simulink model "softLog"  (R2025b)
settings: configuration reference "MCConfiguration" (kept outside this file)
settings Model: DataDictionary=embeddedBoard_common.sldd  OrderFunctionsByDependency=on  Creator=rpumpo  LastModifiedBy=rpumpo
settings ConfigSetRef: SourceName=MCConfiguration

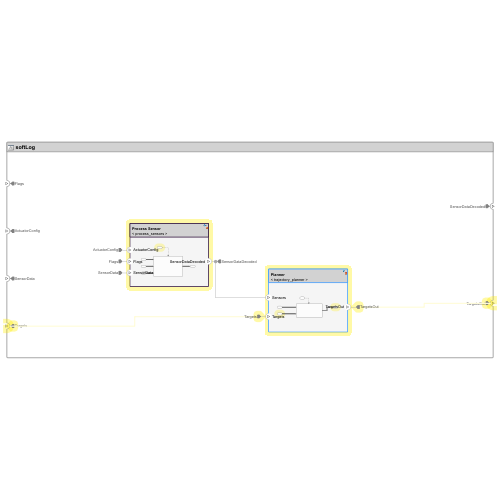
[thumbnail: Simulink's stored preview of the top-level diagram]
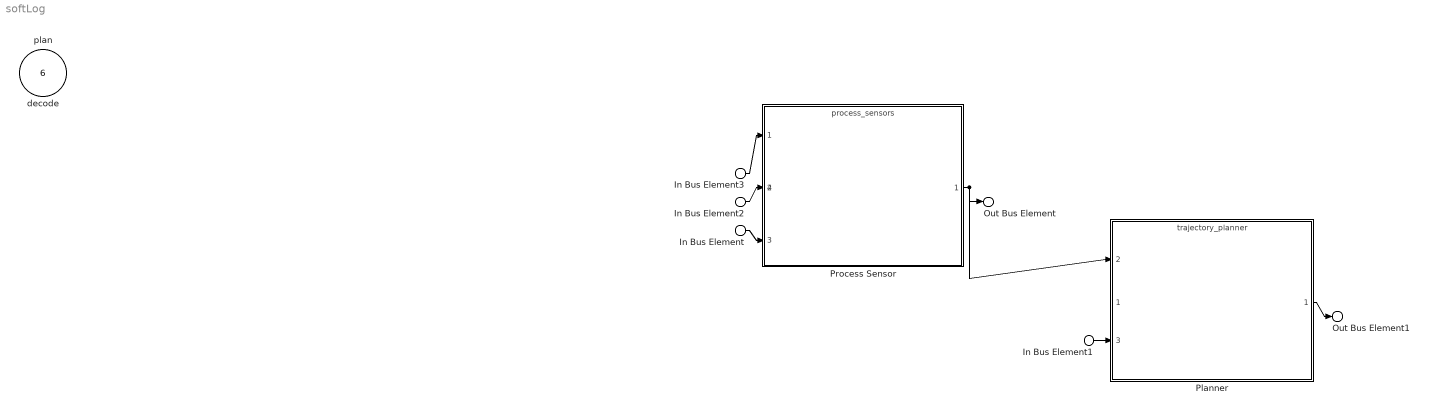
== system softLog ==
  In Bus Element2 : Inport  PortName=Flags
  In Bus Element3 : Inport  Port=2  PortName=ActuatorConfig
  In Bus Element : Inport  Port=3  PortName=SensorData
  In Bus Element1 : Inport  Port=4  PortName=Targets
  decode : Inport  Port=5  OutputFunctionCall=on
  plan : Inport  Port=6  OutputFunctionCall=on
  Planner : ModelReference  ModelNameDialog=trajectory_planner.slx  SimulationMode=Normal  ScheduleRates=on  ModelReferenceVersion=2.99
      settings: PortSchema="{\"entries\":[{\"content\":{\"headerSize\":38,\"margin\":15,\"minimumSpacing\":25,\"sides\":[{\"content\":{\"connectorIds\":[\"In2\",\"In3\"]},\"type\":\"ConnectorPlacement.EquallySpacedRectSide\",\"uuid\":\"5bc97249-f5b2-494b-970a-de3b3bfd1883\"},{\"content\":{\"connectorIds\":[\"Out1\"],\"side\":\"RIGHT\"},\"type\":\"ConnectorPlacement.EquallySpacedRectSide\",\"uuid\":\"c27ffe8a-4f1e-4977-8b42-d9f4b26c99eb\"},{\"content\":{\"side\":\"TOP\"},\"type\":\"ConnectorPlacement.EquallySpacedRectSide\",\"uuid\":\"ea9c3efe-70a2-4d08-a1da-b2e728a33970\"},{\"content\":{\"connectorIds\":[\"In1\"],\"side\":\"HIDDEN\"},\"type\":\"ConnectorPlacement.EquallySpacedRectSide\",\"uuid\":\"de6ac64e-1bcc-4d04-bbff-3f527994b2c1\"}]},\"type\":\"ConnectorPlacement.EquallySpacedConnector\",\"uuid\":\"8d7bebf6-8f7c-4b76-a6d3-5057827f12fc\"}],\"packageUris\":[\"http://schema.mathworks.com/mf0/Connector/R2020b\"],\"version\":\"1.0\"}"
  Process Sensor : ModelReference  ModelNameDialog=process_sensors.slx  SimulationMode=Normal  ScheduleRates=on  ModelReferenceVersion=2.14
      settings: PortSchema="{\"entries\":[{\"content\":{\"headerSize\":38,\"margin\":15,\"minimumSpacing\":25,\"sides\":[{\"content\":{\"connectorIds\":[\"In1\",\"In2\",\"In3\"]},\"type\":\"ConnectorPlacement.EquallySpacedRectSide\",\"uuid\":\"2276003e-9a77-4c7c-a76e-f56f210be786\"},{\"content\":{\"connectorIds\":[\"Out1\"],\"side\":\"RIGHT\"},\"type\":\"ConnectorPlacement.EquallySpacedRectSide\",\"uuid\":\"004a3e19-af23-4274-82b4-d85717ce6563\"},{\"content\":{\"side\":\"TOP\"},\"type\":\"ConnectorPlacement.EquallySpacedRectSide\",\"uuid\":\"ffcf1e21-5ab5-4695-b5dd-709d42365f35\"},{\"content\":{\"connectorIds\":[\"In4\"],\"side\":\"HIDDEN\"},\"type\":\"ConnectorPlacement.EquallySpacedRectSide\",\"uuid\":\"30b5247d-ec6a-4f59-b9c2-740d34c609ee\"}]},\"type\":\"ConnectorPlacement.EquallySpacedConnector\",\"uuid\":\"0f94fc51-6463-431b-bfe7-6597b483019c\"}],\"packageUris\":[\"http://schema.mathworks.com/mf0/Connector/R2020b\"],\"version\":\"1.0\"}"
  Out Bus Element : Outport  PortName=SensorDataDecoded
  Out Bus Element1 : Outport  Port=2  PortName=TargetsOut
  wires:
  In Bus Element2/1 -> Process Sensor/2
  In Bus Element/1 -> Process Sensor/3
  In Bus Element3/1 -> Process Sensor/1
  Process Sensor/1 -> Out Bus Element/1, Planner/2
  Planner/1 -> Out Bus Element1/1
  In Bus Element1/1 -> Planner/3
